simulink model "Bode_01"  (R2021a)
settings: Solver=VariableStepAuto  StartTime=0.0  StopTime=10.0  RelTol=1e-3
libraries: slctrlblks x1
settings Model: Creator=xpess  LastModifiedBy=xpess

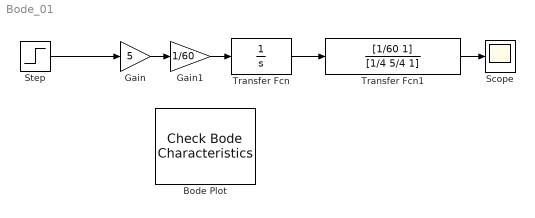
== system Bode_01 ==
  Bode Plot : slctrlblks/Model Verification/Check Bode  Characteristics  InstantiateOnLoad=on  SaveOperatingPoints=off  LinearizationIOs={'/Step', 1, 'in', 'on', '';'/Transfer Fcn1', 1, 'out', 'on', ''}  LinearizeAt=SnapshotTimes  SnapshotTimes=[0]  TriggerType=rising  SampleTime=auto  RateConversionMethod=zoh  PreWarpFreq=10  UseExactDelayModel=off  UseFullBlockNameLabels=off  UseBusSignalLabels=off  enabled=on  stopWhenAssertionFail=off  export=off  ViewDlgPos=[623 143.666666666667 723.333333333333 489.333333333333]  OpenViewOnLoad=on  LaunchViewOnOpen=off  FrequencyUnits=rad/s  MagnitudeUnits=dB  PhaseUnits=deg  TimeUnits=seconds  EnableUpperBound=off  UpperBoundFrequencies=[]  UpperBoundMagnitudes=[]  EnableLowerBound=off  LowerBoundFrequencies=[]  LowerBoundMagnitudes=[]
  Gain : Gain  Gain=5
  Gain1 : Gain  Gain=1/60
  Scope : Scope
  Step : Step  SampleTime=0
  Transfer Fcn : TransferFcn  Denominator=[1 0]
  Transfer Fcn1 : TransferFcn  Numerator=[1/60 1]  Denominator=[1/4 5/4 1]
  wires:
  Step/1 -> Gain/1
  Gain/1 -> Gain1/1
  Gain1/1 -> Transfer Fcn/1
  Transfer Fcn/1 -> Transfer Fcn1/1
  Transfer Fcn1/1 -> Scope/1
